simulink model "hop_zero_aerial"  (R2019a)
settings: Solver=VariableStepAuto  StartTime=0.0  StopTime=ta  RelTol=1e-3
values from neighbouring files (symbols this model uses):
  g = -9.81    [MMR.m]    (also in MMR_alfa0.m; MMR_alone.m; MMR_hop_zero.m = 9.81)
  vyfinal = vy( length(vy) )    [MMR.m]    (also in MMR_alfa0.m; MMR_alone.m; MMR_hop_zero.m)
  yfinal = y( length(y) )    [MMR.m]    (also in MMR_alfa0.m; MMR_alone.m; MMR_hop_zero.m)
settings Model: Creator=Jesus  LastModifiedBy=Jesus

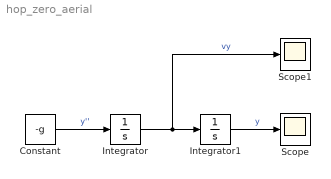
== system hop_zero_aerial ==
  Constant : Constant  Value=-g
  Integrator : Integrator  InitialCondition=vyfinal
  Integrator1 : Integrator  InitialCondition=yfinal
  Scope : Scope
  Scope1 : Scope
  wires:
  Constant/1 -> Integrator/1  "y''"
  Integrator/1 -> Scope1/1, Integrator1/1  "vy"
  Integrator1/1 -> Scope/1  "y"
